simulink library "libconnext"  (R2018a)
settings: Solver=VariableStepAuto  StartTime=0.0  StopTime=10.0  RelTol=1e-3
undefined symbols (not defined in the file): Take
libraries: DDSLibrary x7
settings Model: Creator=Lenovo  LastModifiedBy=Lenovo

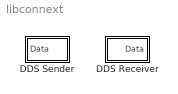
== system libconnext ==
  DDS Sender : Subsystem
  DDS Receiver : Subsystem  mask{domainid=0, topictype=[], topicname=[], sampletime=-1}
      mask prompts: domainid "Domain ID"; topictype "Topic Type"; topicname "Topic Name"; sampletime "Sample Time"

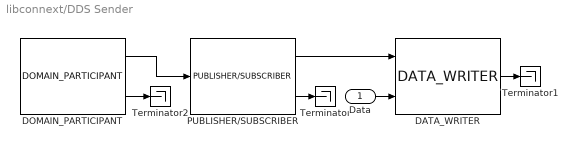
== system libconnext/DDS Sender ==
  Data : Inport
  DATA_WRITER : DDSLibrary/DATA_WRITER  SParam1=ShapeType  SParam2=Circle  SParam3=-1
      settings: SourceProductName=DDS Blockset
  DOMAIN_PARTICIPANT : DDSLibrary/DOMAIN_PARTICIPANT  SParam3=0  SParam1=-1  PeerIPList=[]
      settings: SourceProductName=DDS Blockset
  PUBLISHER/SUBSCRIBER : DDSLibrary/PUBLISHER//SUBSCRIBER  SParam2=Subscriber  SParam1=-1
      settings: SourceProductName=DDS Blockset
  Terminator : Terminator
  Terminator1 : Terminator
  Terminator2 : Terminator
  wires:
  DOMAIN_PARTICIPANT/1 -> PUBLISHER/SUBSCRIBER/1
  Data/1 -> DATA_WRITER/2
  PUBLISHER/SUBSCRIBER/1 -> DATA_WRITER/1
  DATA_WRITER/1 -> Terminator1/1
  DOMAIN_PARTICIPANT/2 -> Terminator2/1
  PUBLISHER/SUBSCRIBER/2 -> Terminator/1

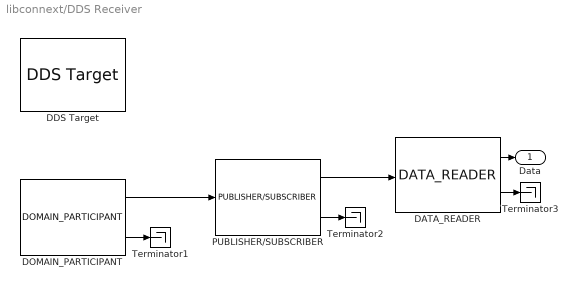
== system libconnext/DDS Receiver ==
  DATA_READER : DDSLibrary/DATA_READER  SParam2=ShapeType  SParam3=Circle  SParam4=-1  SParam11=off  SParam1=off  SParam6=2  SParam7=Take()  SParam8=No Filter  SParam9='x > %0 and x < %1'  SParam10={'5', '123'}
      settings: SourceProductName=DDS Blockset
  DDS Target : DDSLibrary/DDS Target  SParam1=RTI Connext DDS  SParam2=Static  SParam3=Dynamic  SampleTime=-1  LocalIPAddress=30.30.30.1  LocalIPSubnet=255.255.255.0
      settings: SourceProductName=DDS Blockset
  DOMAIN_PARTICIPANT : DDSLibrary/DOMAIN_PARTICIPANT  SParam3=domainid  SParam1=sampletime  PeerIPList=[]
      settings: SourceProductName=DDS Blockset
  PUBLISHER/SUBSCRIBER : DDSLibrary/PUBLISHER//SUBSCRIBER  SParam2=Subscriber  SParam1=-1
      settings: SourceProductName=DDS Blockset
  Terminator1 : Terminator
  Terminator2 : Terminator
  Terminator3 : Terminator
  Data : Outport
  wires:
  DATA_READER/1 -> Data/1
  DOMAIN_PARTICIPANT/1 -> PUBLISHER/SUBSCRIBER/1
  PUBLISHER/SUBSCRIBER/1 -> DATA_READER/1
  PUBLISHER/SUBSCRIBER/2 -> Terminator2/1
  DATA_READER/2 -> Terminator3/1
  DOMAIN_PARTICIPANT/2 -> Terminator1/1
